simulink library "pbe"  (Simulink 8.1)
settings: Solver=ode1  StartTime=0.0  StopTime=Inf  FixedStep=0.001  RelTol=1e-3
PostLoadFcn:
  | , if any(exist('dsrtsu_mdlpostloadfcn', 'file') == [2, 3, 6]), try dsrtsu_mdlpostloadfcn('Execute', bdroot); catch fprintf('Error in PostLoadFcn (dsrtsu_mdlpostloadfcn) for model "%s":\n %s\n', bdroot, lasterr); end, end,
undefined symbols (not defined in the file or in its folder): KACC_ACCBrakeDisableSpd_kph, KACC_BrakeRelMinSpd_kph
libraries: hcu_lib x2, bsd x1, bsg x1, btd x1, btg x1
settings Model: DSRTSU_INTERNAL_RTI_VER=450  DSRTSU_INTERNAL_RTI_TYPE=rti1401  RTICANMMDATA=struct('GeneralSetupData',struct('modelroot','D:\ELN150201_TAIWAN\trunk\AdasDragon\software\sw_development\arch\app\acc','generalsettings',struct('filesettings',struct('destfolder',struct('Name','RTICANMM_FILES','Check',1),'buildfolder',struct('Name','.','Check',1),'AbsDestfolder',struct('Name','D:\ELN150201_TAIWAN\trunk\AdasDragon\software\sw_development\arch\app\acc\RTICANMM_FILES'),'AbsBuildfolder',struct('Name','D:\ELN150201_TAIWAN\trunk\AdasDragon\software\sw_development\arch\app\acc'))),'options',struct('addpaths',1,'rmpaths',1,'addtrcexclusion',logical(1),'cannavigator',struct('checkmonitoring',0),'show_usrtrc',0,'use_usrtrc',0),'advanced',struct('options',[1 1 1 1 1 1 1 1 1 1 1 1 1 1 1 1 1 1 1 1 1 1 1 1 1 1 1 1 1 1 1 1 1 1 1 1 1 1 1 1 1 1 1 1 1 1 1 1 1 1 1 1 1 1 1 1 1 1 1 1 1 1 1 1 1 1 1 1 1 1 1 1 1 1 1 1 1 1 1 1 1 1 1 1 1 1 1 1 1 1 1 1 1 1 1 1 1 1 1 1]),'MPSetup',{{}},'modelname','pbe','block','pbe'))  DSRTSU_INTERNAL_RTIFPGA=40  Creator=AT015555  LastModifiedBy=AT015555

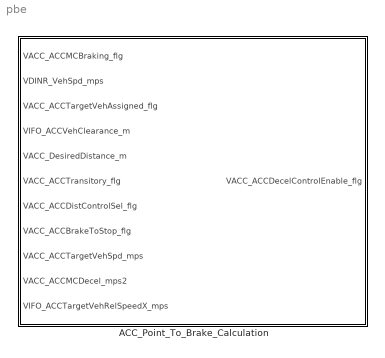
== system pbe ==
  ACC_Point_To_Brake_Calculation : Subsystem

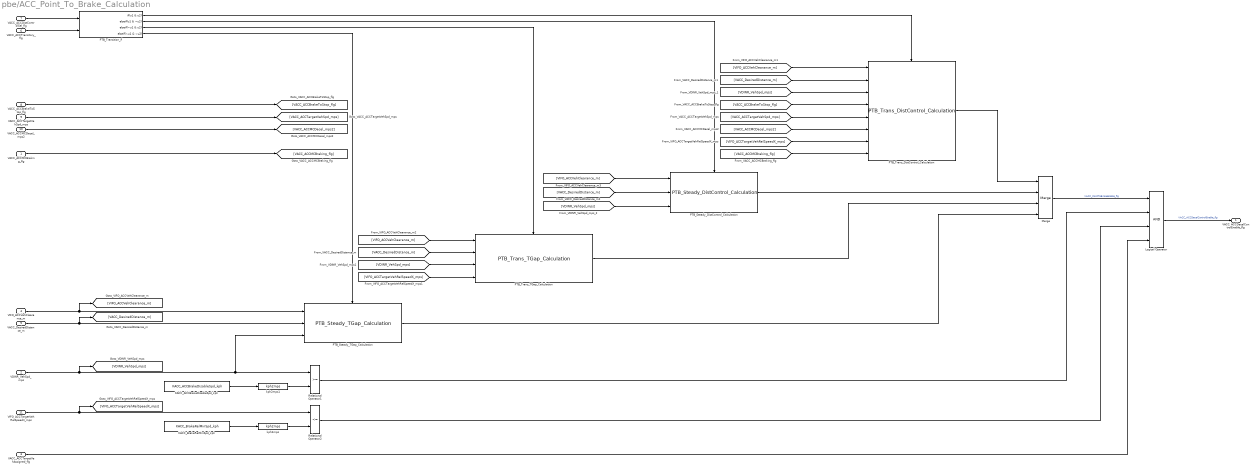
== system pbe/ACC_Point_To_Brake_Calculation ==
  VACC_ACCMCBraking_flg : Inport
  VDINR_VehSpd_mps : Inport  Port=2
  VACC_ACCTargetVehAssigned_flg : Inport  Port=3
  VIFO_ACCVehClearance_m : Inport  Port=4
  VACC_DesiredDistance_m : Inport  Port=5
  VACC_ACCTransitory_flg : Inport  Port=6
  VACC_ACCDistControlSel_flg : Inport  Port=7
  VACC_ACCBrakeToStop_flg : Inport  Port=8
  VACC_ACCTargetVehSpd_mps : Inport  Port=9
  VACC_ACCMCDecel_mps2 : Inport  Port=10
  VIFO_ACCTargetVehRelSpeedX_mps : Inport  Port=11
  KACC_ACCBrakeDisableSpd_kph : Constant  Value=KACC_ACCBrakeDisableSpd_kph
  KACC_BrakeRelMinSpd_kph : Constant  Value=KACC_BrakeRelMinSpd_kph
  Logical Operator : Logic  Inputs=4  AllPortsSameDT=off  OutDataTypeStr=boolean
  Merge : Merge  Inputs=4
  PTB_Steady_DistControl_Calculation : bsd/PTB_Steady_DistControl_Calculation
  PTB_Steady_TGap_Calculation : bsg/PTB_Steady_TGap_Calculation
  PTB_Trans_DistControl_Calculation : btd/PTB_Trans_DistControl_Calculation
  PTB_Trans_TGap_Calculation : btg/PTB_Trans_TGap_Calculation
  PTB_Transition_if : If  NumInputs=2  IfExpression=u1 & u2  ElseIfExpressions=u1 & ~u2, ~u1 & u2, ~u1 & ~u2  ShowElse=off
  Relational Operator1 : RelationalOperator  OutDataTypeStr=boolean
  Relational Operator2 : RelationalOperator  Operator=<=  OutDataTypeStr=boolean
  kph2mps : hcu_lib/kph2mps
  kph2mps1 : hcu_lib/kph2mps
  VACC_ACCDecelControlEnable_flg : Outport
  wires:
  Logical Operator/1 -> VACC_ACCDecelControlEnable_flg/1  "VACC_ACCDecelControlEnable_flg"
  VACC_ACCDistControlSel_flg/1 -> PTB_Transition_if/1
  VACC_ACCTransitory_flg/1 -> PTB_Transition_if/2
  VACC_DesiredDistance_m/1 -> PTB_Steady_TGap_Calculation/2, [VACC_DesiredDistance_m]
  VIFO_ACCVehClearance_m/1 -> [VIFO_ACCVehClearance_m], PTB_Steady_TGap_Calculation/1
  PTB_Transition_if/1 -> PTB_Trans_DistControl_Calculation/Action
  [VIFO_ACCVehClearance_m] -> PTB_Trans_TGap_Calculation/1
  [VACC_DesiredDistance_m] -> PTB_Trans_TGap_Calculation/2
  VIFO_ACCTargetVehRelSpeedX_mps/1 -> Relational Operator2/1, [VIFO_ACCTargetVehRelSpeedX_mps]
  PTB_Transition_if/3 -> PTB_Trans_TGap_Calculation/Action
  PTB_Transition_if/4 -> PTB_Steady_TGap_Calculation/Action
  [VIFO_ACCVehClearance_m] -> PTB_Trans_DistControl_Calculation/1
  [VACC_DesiredDistance_m] -> PTB_Trans_DistControl_Calculation/2
  VDINR_VehSpd_mps/1 -> [VDINR_VehSpd_mps], PTB_Steady_TGap_Calculation/3, Relational Operator1/1
  PTB_Trans_DistControl_Calculation/1 -> Merge/1
  PTB_Trans_TGap_Calculation/1 -> Merge/3
  PTB_Steady_TGap_Calculation/1 -> Merge/4
  [VDINR_VehSpd_mps] -> PTB_Trans_DistControl_Calculation/3
  PTB_Steady_DistControl_Calculation/1 -> Merge/2
  PTB_Transition_if/2 -> PTB_Steady_DistControl_Calculation/Action
  [VDINR_VehSpd_mps] -> PTB_Steady_DistControl_Calculation/3
  [VACC_DesiredDistance_m] -> PTB_Steady_DistControl_Calculation/2
  [VIFO_ACCVehClearance_m] -> PTB_Steady_DistControl_Calculation/1
  [VIFO_ACCTargetVehRelSpeedX_mps] -> PTB_Trans_DistControl_Calculation/7
  Relational Operator2/1 -> Logical Operator/3
  [VIFO_ACCTargetVehRelSpeedX_mps] -> PTB_Trans_TGap_Calculation/4
  KACC_ACCBrakeDisableSpd_kph/1 -> kph2mps1/1
  Relational Operator1/1 -> Logical Operator/2
  KACC_BrakeRelMinSpd_kph/1 -> kph2mps/1
  kph2mps/1 -> Relational Operator2/2
  [VDINR_VehSpd_mps] -> PTB_Trans_TGap_Calculation/3
  Merge/1 -> Logical Operator/1  "VACC_PointToBrakeEnable_flg"
  VACC_ACCTargetVehAssigned_flg/1 -> Logical Operator/4
  VACC_ACCBrakeToStop_flg/1 -> [VACC_ACCBrakeToStop_flg]
  [VACC_ACCBrakeToStop_flg] -> PTB_Trans_DistControl_Calculation/4
  VACC_ACCTargetVehSpd_mps/1 -> [VACC_ACCTargetVehSpd_mps]
  [VACC_ACCTargetVehSpd_mps] -> PTB_Trans_DistControl_Calculation/5
  VACC_ACCMCDecel_mps2/1 -> [VACC_ACCMCDecel_mps2]
  [VACC_ACCMCDecel_mps2] -> PTB_Trans_DistControl_Calculation/6
  VACC_ACCMCBraking_flg/1 -> [VACC_ACCMCBraking_flg]
  [VACC_ACCMCBraking_flg] -> PTB_Trans_DistControl_Calculation/8
  kph2mps1/1 -> Relational Operator1/2
